simulink model "Missile_Trim"  (R2018b)
settings: Solver=ode4  StartTime=0.0  StopTime=5  FixedStep=Step_Size  RelTol=1e-3  EnableMultiTasking=on
values from neighbouring files (symbols this model uses):
  Alt_Trim = altitude_range(i)    [Missile_Trim_Main.m]    (also in Trim_Solution_a.mat = 0)
  D = 0.150    (= 0.15)    [Missile_Data.m]
  G_Turn = Turn_dot_Trim * Speed_Trim / UNIT_GRAV    [Missile_Trim_Main.m]
  Gamma_Trim = 0.0 * UNIT_DEG2RAD    [Missile_Trim_Main.m]
  Init_Cnstr1 = 0.0    (= 0)    [Missile_Trim_Main.m]
  Init_Cnstr2 = 0.0    (= 0)    [Missile_Trim_Main.m]
  Init_Cnstr3 = 0.0    (= 0)    [Missile_Trim_Main.m]
  Mass = 30.0    (= 30)    [Missile_Data.m]
  S = ( pi / 4 ) * D^2    (= 0.0176714586764)    [Missile_Data.m]
  Speed_Trim = Mach_Trim*interp1(ALT,SOS_Table,Alt_Trim)    [Missile_Trim_Main.m]
  Tbl_ALPHAT = [ 0     4     8    12    16 ]    [Missile_Data.m]
  Tbl_CL_ALPHAT = [ -0.0988   -0.4859   -0.5870   -0.4802   -0.3334   -0.0210 ]    [Missile_Data.m]
  Tbl_CL_DEL_R = [ 5.2712    5.7640    6.1650    6.6234    7.1963    8.4110 ]    [Missile_Data.m]
  Tbl_CL_P = [ -17.9516  -19.6297  -20.9956  -22.5566  -24.5079  -28.6446 ]    [Missile_Data.m]
  Tbl_CM_0 = [ 0   -2.2250   -3.9280   -4.8580   -5.6940 ... (first row only)    [Missile_Data.m]
  Tbl_CM_DEL_P = [ -20.7182  -22.5631  -23.6059  -24.7632  -26.1269  -29.5646 ]    [Missile_Data.m]
  Tbl_CM_PHIT = [ 0   -0.0024   -0.0898   -0.2360   -0.3546 ... (first row only)    [Missile_Data.m]
  Tbl_CM_Q = [ -82.9643  -47.4409  -32.7732  -16.7304  -43.2010  -56.1499 ]    [Missile_Data.m]
  Tbl_CN_DEL_Y = [ -0.3616   -0.3938   -0.4120   -0.4322   -0.4560   -0.5160 ]    [Missile_Data.m]
  Tbl_CN_PHIT = [ 0    0.0040    0.0098    0.1116    0.3049 ... (first row only)    [Missile_Data.m]
  Tbl_CN_R = [ -82.9643  -47.4409  -32.7732  -16.7304  -43.2010  -56.1499 ]    [Missile_Data.m]
  Tbl_CX_0 = [ -0.3840   -0.3670   -0.3550   -0.3460   -0.3390   -0.3410 ]    [Missile_Data.m]
  Tbl_CX_ALPHAT = [ 0.0788    0.0752    0.0680    0.0573    0.0573    0.0573 ]    [Missile_Data.m]
  Tbl_CX_DEL_EFF = [ -16.8080  -17.8585  -18.9090  -19.9595  -20.4847  -23.1110 ]    [Missile_Data.m]
  Tbl_CY_DEL_Y = [ 5.3056    5.7754    6.0504    6.3484    6.6921    7.5745 ]    [Missile_Data.m]
  Tbl_CY_PHIT = [ 0    0.0070    0.0819    0.2313    0.2992 ... (first row only)    [Missile_Data.m]
  Tbl_CZ_0 = [ 0   -2.0680   -3.9700   -5.4250   -6.6810 ... (first row only)    [Missile_Data.m]
  Tbl_CZ_DEL_P = [ -5.3056   -5.7754   -6.0504   -6.3484   -6.6921   -7.5745 ]    [Missile_Data.m]
  Tbl_CZ_PHIT = [ 0    0.0089    0.1842    0.3041    0.2039 ... (first row only)    [Missile_Data.m]
  Tbl_MACH = [ 0.2    0.3    0.4    0.5    0.6    0.7 ]    [Missile_Data.m]
  Theta_dot_Trim = 0.0 * UNIT_DEG2RAD    [Missile_Trim_Main.m]
  Turn_dot_Trim = 0.0 * UNIT_DEG2RAD    [Missile_Trim_Main.m]
  XCG = 0.809    [Missile_Data.m]
  XREF = 0.809    [Missile_Data.m]
undefined symbols (not defined in the file or in its folder): ALT, Init_Euler, Init_Rate, Init_Vel, SOS_Table, UNIT_GRAV
libraries: simulink_extras x6, aerolibtransform2 x4, aerolibasang x3, UAS_Model_library x2, shared6dofsys x2, sharedtransform x1, sharedutil x1, shared6dof x1
settings Model: Creator=e803534  LastModifiedBy=auten
settings OptimizationCC: LifeSpan=inf
settings DebuggingCC: LibraryContextMissingDiagnostic=none  SFUnexpectedBacktrackingDiag=warning  SFNoUnconditionalDefaultTransitionDiag=warning  SFExecutionAtInitializationDiag=none
settings SFSimCC: SimUseLocalCustomCode=off
settings RTWCC: RTWUseLocalCustomCode=off
settings CodeAppCC: StateflowObjectComments=on
settings GRTTargetCC: TargetLangStandard=C89/C90 (ANSI)  GeneratePreprocessorConditionals=Disable all
settings ConfigComp: CovMetricSettings=dw  CovHtmlReporting=on  CovSaveCumulativeToWorkspaceVar=on  CovSaveSingleToWorkspaceVar=on  CovExternalEMLEnable=off

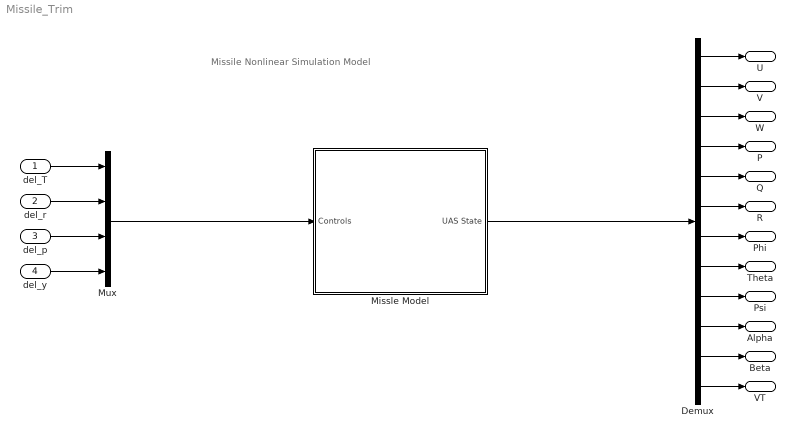
== system Missile_Trim ==
  note: Missile Nonlinear Simulation Model
  del_T : Inport
  "del_r " : Inport  Port=2
  del_p : Inport  Port=3
  del_y : Inport  Port=4
  Demux : Demux  Outputs=12
  Missle Model : Subsystem
  Mux : Mux
  U : Outport
  V : Outport  Port=2
  W : Outport  Port=3
  P : Outport  Port=4
  Q : Outport  Port=5
  R : Outport  Port=6
  Phi : Outport  Port=7
  Theta : Outport  Port=8
  Psi : Outport  Port=9
  Alpha : Outport  Port=10
  Beta : Outport  Port=11
  VT : Outport  Port=12
  wires:
  Mux/1 -> Missle Model/1(Controls)
  del_p/1 -> Mux/3
  "del_r "/1 -> Mux/2
  del_T/1 -> Mux/1
  del_y/1 -> Mux/4
  Missle Model/1(UAS State) -> Demux/1
  Demux/1 -> U/1
  Demux/3 -> W/1
  Demux/5 -> Q/1
  Demux/6 -> R/1
  Demux/7 -> Phi/1
  Demux/9 -> Psi/1
  Demux/10 -> Alpha/1
  Demux/11 -> Beta/1
  Demux/12 -> VT/1
  Demux/4 -> P/1
  Demux/2 -> V/1
  Demux/8 -> Theta/1

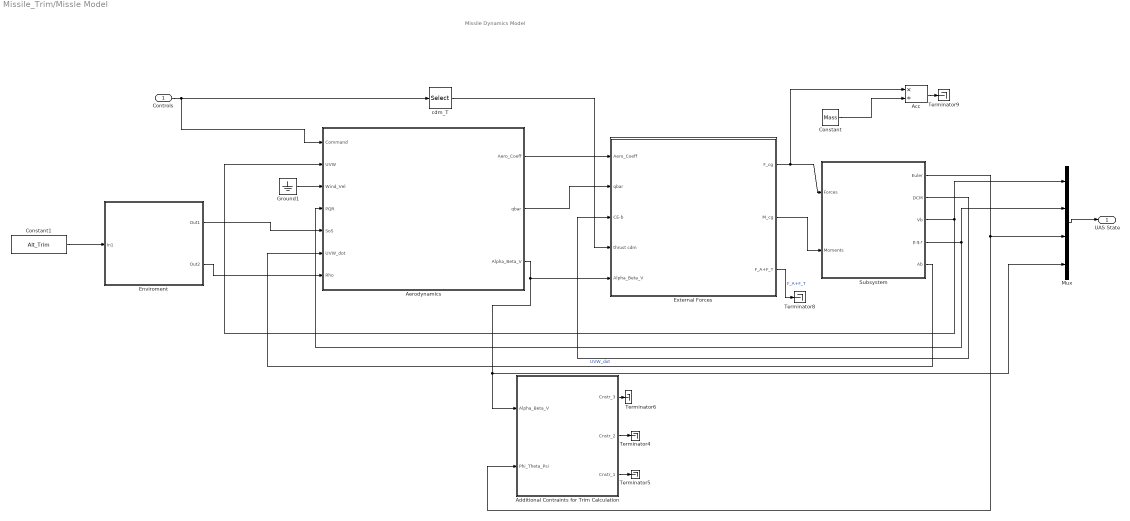
== system Missile_Trim/Missle Model ==
  note: Missile Dynamics Model
  Controls : Inport
  Acc : Product  Inputs=*/  RndMeth=Zero
  Additional Contraints for Trim Calculation : Subsystem
  Aerodynamics : Subsystem
  Constant : Constant  Value=Mass
  Constant1 : Constant  Value=Alt_Trim
  Enviroment : Subsystem
  External Forces : Subsystem
  Ground1 : Ground
  Mux : Mux
  Subsystem : Subsystem
  Terminator{4..6,8..9} (5 alike) : Terminator
  cdm_T : Selector  InputPortWidth=4  IndexOptions=Index vector (dialog)  Indices=[1]  OutputSizes=1
  UAS State : Outport
  wires:
  Controls/1 -> Aerodynamics/1(Command), cdm_T/1
  External Forces/1(F_cg) -> Subsystem/1(Forces), Acc/1
  External Forces/2(M_cg) -> Subsystem/2(Moments)
  Constant/1 -> Acc/2
  Mux/1 -> UAS State/1
  Subsystem/3(Vb) -> Mux/1, Aerodynamics/2(UVW)
  Subsystem/4(p,q,r) -> Aerodynamics/4(PQR), Mux/2
  Acc/1 -> Terminator9/1
  Additional Contraints for Trim Calculation/2(Cnstr_2) -> Terminator4/1
  Additional Contraints for Trim Calculation/3(Cnstr_1) -> Terminator5/1
  Additional Contraints for Trim Calculation/1(Cnstr_3) -> Terminator6/1
  Subsystem/1(Euler) -> Mux/3, Additional Contraints for Trim Calculation/2(Phi_Theta_Psi)
  Subsystem/2(DCM) -> External Forces/3(CE-b)
  cdm_T/1 -> External Forces/4(thrust cdm)
  External Forces/3(F_A+F_T) -> Terminator8/1  "F_A+F_T"
  Aerodynamics/3(Alpha_Beta_V) -> Additional Contraints for Trim Calculation/1(Alpha_Beta_V), Mux/4, External Forces/5(Alpha_Beta_V)
  Ground1/1 -> Aerodynamics/3(Wind_Vel)
  Subsystem/5(Ab) -> Aerodynamics/6(UVW_dot)  "UVW_dot"
  Aerodynamics/1(Aero_Coeff) -> External Forces/1(Aero_Coeff)
  Aerodynamics/2(qbar) -> External Forces/2(qbar)
  Constant1/1 -> Enviroment/1(In1)
  Enviroment/1(Out1) -> Aerodynamics/5(SoS)
  Enviroment/2(Out2) -> Aerodynamics/7(Rho)

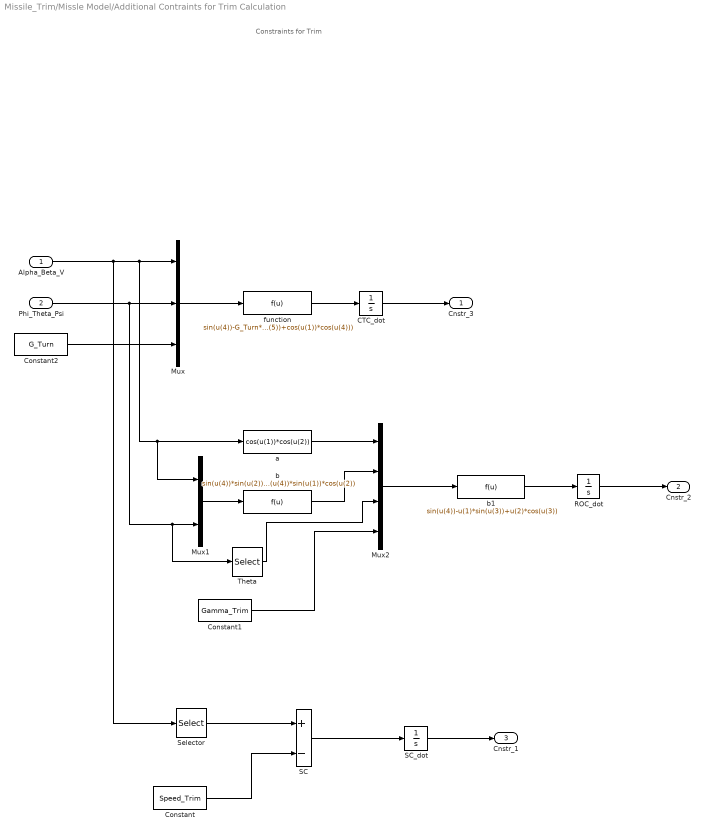
== system Missile_Trim/Missle Model/Additional Contraints for Trim Calculation ==
  note: Constraints for Trim
  Alpha_Beta_V : Inport  PortDimensions=3
  Phi_Theta_Psi : Inport  Port=2  PortDimensions=3
  CTC_dot : Integrator  InitialCondition=Init_Cnstr3
  Constant : Constant  Value=Speed_Trim
  Constant1 : Constant  Value=Gamma_Trim
  Constant2 : Constant  Value=G_Turn
  Mux : Mux  Inputs=3
  Mux1 : Mux  Inputs=2
  Mux2 : Mux
  ROC_dot : Integrator  InitialCondition=Init_Cnstr2
  SC : Sum  Inputs=+-
  SC_dot : Integrator  InitialCondition=Init_Cnstr1
  Selector : Selector  InputPortWidth=3  IndexOptions=Index vector (dialog)  Indices=[3]  OutputSizes=1
  Theta : Selector  InputPortWidth=3  IndexOptions=Index vector (dialog)  Indices=[2]  OutputSizes=1
  a : Fcn  Expr=cos(u(1))*cos(u(2))
  b : Fcn  Expr=sin(u(4))*sin(u(2))+cos(u(4))*sin(u(1))*cos(u(2))
  b1 : Fcn  Expr=sin(u(4))-u(1)*sin(u(3))+u(2)*cos(u(3))
  function : Fcn  Expr=sin(u(4))-G_Turn*cos(u(2))*(sin(u(1))*tan(u(5))+cos(u(1))*cos(u(4)))
  Cnstr_3 : Outport
  Cnstr_2 : Outport  Port=2
  Cnstr_1 : Outport  Port=3
  wires:
  CTC_dot/1 -> Cnstr_3/1
  Alpha_Beta_V/1 -> Selector/1, Mux1/1, a/1, Mux/1
  Phi_Theta_Psi/1 -> Theta/1, Mux1/2, Mux/2
  Constant2/1 -> Mux/3
  Mux/1 -> function/1
  function/1 -> CTC_dot/1
  Mux1/1 -> b/1
  b/1 -> Mux2/2
  a/1 -> Mux2/1
  Constant1/1 -> Mux2/4
  Theta/1 -> Mux2/3
  Mux2/1 -> b1/1
  ROC_dot/1 -> Cnstr_2/1
  b1/1 -> ROC_dot/1
  SC_dot/1 -> Cnstr_1/1
  Selector/1 -> SC/1
  Constant/1 -> SC/2
  SC/1 -> SC_dot/1

== system Missile_Trim/Missle Model/Aerodynamics ==
  Command : Inport
  UVW : Inport  Port=2
  Wind_Vel : Inport  Port=3
  PQR : Inport  Port=4
  SoS : Inport  Port=5
  UVW_dot : Inport  Port=6
  Rho : Inport  Port=7
  Aerodynanamic Coefficents : Subsystem
  Wind-axes Velocitie : Subsystem  AncestorBlock=UAS_Model_library/External Forces/Aerodynamics/Wind-axes Velocitie
  Aero_Coeff : Outport
  qbar : Outport  Port=2
  Alpha_Beta_V : Outport  Port=3
  wires:
  SoS/1 -> Wind-axes Velocitie/3(SoS)
  UVW/1 -> Wind-axes Velocitie/1(UVW)
  Aerodynanamic Coefficents/1(Aero_Coeff) -> Aero_Coeff/1
  Wind-axes Velocitie/1(Alpha_Beta_V) -> Alpha_Beta_V/1, Aerodynanamic Coefficents/2(Alpha_Beta_V)  "Alpha_Beta_V"
  Wind-axes Velocitie/3(qbar) -> qbar/1
  Wind-axes Velocitie/2(Mach) -> Aerodynanamic Coefficents/3(Mach)
  UVW_dot/1 -> Wind-axes Velocitie/5(UVW_dot)
  PQR/1 -> Aerodynanamic Coefficents/4(PQR), Wind-axes Velocitie/6(PQR)
  Rho/1 -> Wind-axes Velocitie/4(Rho)
  Wind_Vel/1 -> Wind-axes Velocitie/2(Wind_Vel)
  Command/1 -> Aerodynanamic Coefficents/1(Command)

== system Missile_Trim/Missle Model/Enviroment ==
  In1 : Inport
  1-D Lookup Table : Lookup_n-D  NumberOfTableDimensions=1  BreakpointsForDimension1=ALT  Table=SOS_Table  InternalRulePriority=Speed  RndMeth=Simplest  InputSameDT=on
  Atmosphere Model : UAS_Model_library/Envrionment/Atmosphere Model  SystemSampleTime=-1
  Terminator2 : Terminator
  Out1 : Outport
  Out2 : Outport  Port=2
  wires:
  In1/1 -> Atmosphere Model/1, 1-D Lookup Table/1
  Atmosphere Model/1 -> Terminator2/1
  Atmosphere Model/2 -> Out2/1
  1-D Lookup Table/1 -> Out1/1

== system Missile_Trim/Missle Model/External Forces ==
  Aero_Coeff : Inport
  qbar : Inport  Port=2
  CE-b : Inport  Port=3
  thrust cdm : Inport  Port=4
  Alpha_Beta_V : Inport  Port=5
  Aerodynamic Force & Moment : Subsystem  AncestorBlock=UAS_Model_library/External Forces/Aerodynamics/Aerodynamic Force & Moment
  Propulsive Force & Moment : Subsystem  AncestorBlock=UAS_Model_library/External Forces/Propulsive/Propulsive Force & Moment
  Sum of Aerodynamic and Propulsion Forces : Sum
  Total Force & Moment : Subsystem  AncestorBlock=UAS_Model_library/External Forces/Total Force & Moment
  F_cg : Outport
  M_cg : Outport  Port=2
  F_A+F_T : Outport  Port=3
  wires:
  Total Force & Moment/2(M_cg) -> M_cg/1
  Aerodynamic Force & Moment/2(M_aero) -> Total Force & Moment/2(M_aero)
  Propulsive Force & Moment/2(M_prop) -> Total Force & Moment/4(M_prop)
  Total Force & Moment/1(F_cg) -> F_cg/1
  Aerodynamic Force & Moment/1(F_aero) -> Sum of Aerodynamic and Propulsion Forces/1, Total Force & Moment/1(F_aero)
  Propulsive Force & Moment/1(F_prop) -> Sum of Aerodynamic and Propulsion Forces/2, Total Force & Moment/3(F_prop)
  qbar/1 -> Aerodynamic Force & Moment/2(qbar)
  Aero_Coeff/1 -> Aerodynamic Force & Moment/1(Aero_Coeff)
  Sum of Aerodynamic and Propulsion Forces/1 -> F_A+F_T/1
  CE-b/1 -> Total Force & Moment/5("cE-B ")
  thrust cdm/1 -> Propulsive Force & Moment/1(Controls)
  Alpha_Beta_V/1 -> ?

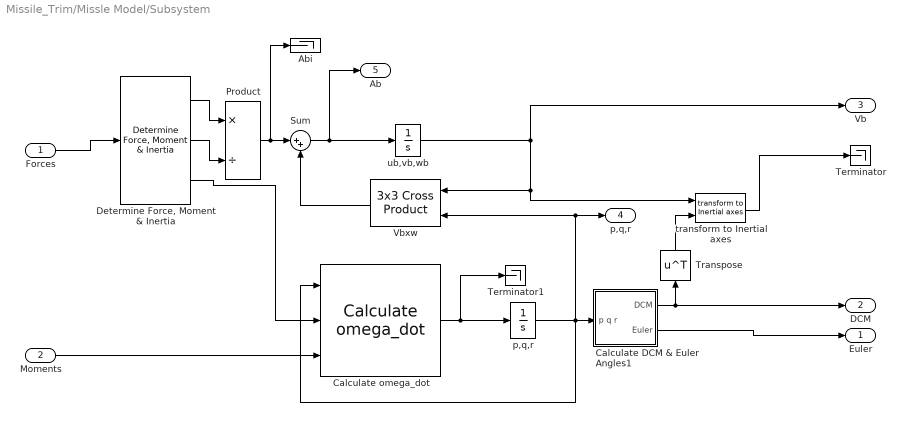
== system Missile_Trim/Missle Model/Subsystem ==
  Forces : Inport  Unit=N  PortDimensions=3
  Moments : Inport  Port=2  Unit=N*m  PortDimensions=3
  Abi : Terminator
  Calculate DCM & Euler Angles1 : Subsystem
  Calculate omega_dot : shared6dofsys/Calculate omega_dot  aMode=aMode
      settings: SourceProductName=Aerospace Blockset  SourceProductBaseCode=AE
  "Determine Force, Moment & Inertia" : UAS_Model_library/Equations of Motion/Determine Force, Moment & Inertia  SystemSampleTime=-1
  Product : Product  Inputs=*/  SaturateOnIntegerOverflow=on  OutDataTypeStr=Inherit: Same as first input
  Sum : Sum  Inputs=|++  SaturateOnIntegerOverflow=on
  Terminator : Terminator
  Terminator1 : Terminator
  Transpose : Math  Operator=transpose  SaturateOnIntegerOverflow=on
  Vbxw : sharedutil/3x3 Cross Product  aMode=aMode
      settings: SourceProductBaseCode=AE
  "p,q,r " : Integrator  InitialCondition=Init_Rate
  "transform to Inertial axes " : shared6dof/6DOF (Euler Angles)/transform to Inertial axes   SystemSampleTime=-1
      settings: SourceProductName=Aerospace Blockset  SourceProductBaseCode=AE
  ub,vb,wb : Integrator  InitialCondition=Init_Vel
  Euler : Outport  Unit=rad
  DCM : Outport  Port=2  Unit=1
  Vb : Outport  Port=3  Unit=m/s
  p,q,r : Outport  Port=4  Unit=rad/s
  Ab : Outport  Port=5  Unit=m/s^2
  wires:
  "transform to Inertial axes "/1 -> Terminator/1
  Calculate omega_dot/1 -> Terminator1/1, "p,q,r "/1
  Sum/1 -> ub,vb,wb/1, Ab/1
  Vbxw/1 -> Sum/2
  Product/1 -> Sum/1, Abi/1
  "p,q,r "/1 -> Calculate DCM & Euler Angles1/1("p q r "), Calculate omega_dot/1, p,q,r/1, Vbxw/2
  Forces/1 -> "Determine Force, Moment & Inertia"/1
  ub,vb,wb/1 -> Vb/1, "transform to Inertial axes "/1, Vbxw/1
  "Determine Force, Moment & Inertia"/2 -> Product/2
  Moments/1 -> Calculate omega_dot/3
  Calculate DCM & Euler Angles1/2(Euler) -> Euler/1
  Calculate DCM & Euler Angles1/1(DCM) -> Transpose/1, DCM/1
  "Determine Force, Moment & Inertia"/3 -> Calculate omega_dot/2
  Transpose/1 -> "transform to Inertial axes "/2
  "Determine Force, Moment & Inertia"/1 -> Product/1

== system Missile_Trim/Missle Model/Aerodynamics/Aerodynanamic Coefficents ==
  Command : Inport
  Alpha_Beta_V : Inport  Port=2
  Mach : Inport  Port=3
  PQR : Inport  Port=4
  Aerodynamics : Subsystem
  del_r del_p del_y : Selector  InputPortWidth=4  IndexOptions=Index vector (dialog)  Indices=[2 3 4]  OutputSizes=1
  delta_eff : Subsystem
  total angle of AoA and Roll : Subsystem
  Aero_Coeff : Outport
  wires:
  del_r del_p del_y/1 -> Aerodynamics/3(control inputs), delta_eff/1(controll)
  total angle of AoA and Roll/2(phi_t) -> Aerodynamics/5(phi_t)
  delta_eff/1(delta_eff) -> Aerodynamics/2(delta_eff)
  Alpha_Beta_V/1 -> total angle of AoA and Roll/1(alpha_beta_V), Aerodynamics/6(alpha_beta_V)
  Command/1 -> del_r del_p del_y/1
  total angle of AoA and Roll/1(alpha_t) -> Aerodynamics/4(alpha_t)
  PQR/1 -> Aerodynamics/7(PQR)
  Aerodynamics/1(Aero_Coeff) -> Aero_Coeff/1
  Mach/1 -> Aerodynamics/1(Mach Number)

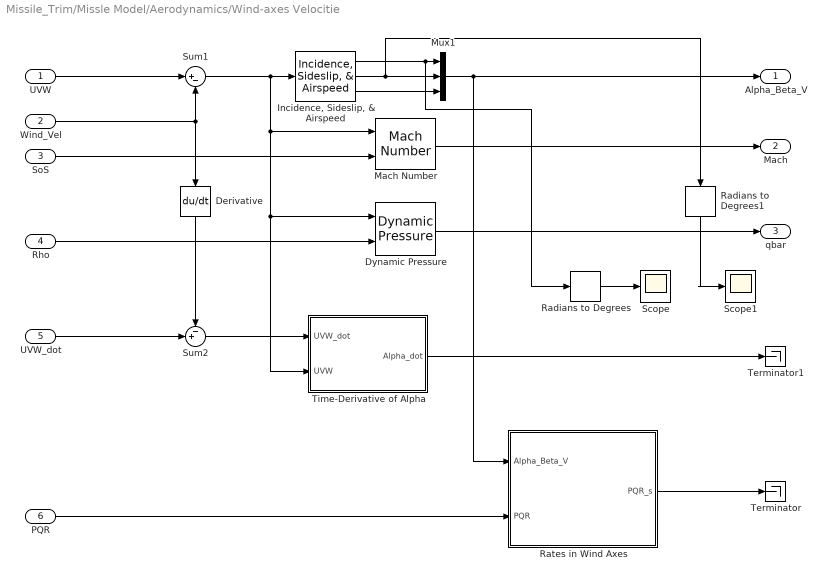
== system Missile_Trim/Missle Model/Aerodynamics/Wind-axes Velocitie ==
  UVW : Inport
  Wind_Vel : Inport  Port=2
  SoS : Inport  Port=3
  Rho : Inport  Port=4
  UVW_dot : Inport  Port=5
  PQR : Inport  Port=6
  Derivative : Derivative
  Dynamic Pressure : aerolibasang/Dynamic Pressure
  "Incidence, Sideslip, & Airspeed" : aerolibasang/Incidence, Sideslip, & Airspeed
      settings: SourceProductName=Aerospace Blockset
  Mach Number : aerolibasang/Mach Number
      settings: SourceProductName=Aerospace Blockset  SourceProductBaseCode=AE
  Mux1 : Mux  Inputs=3
  Radians to Degrees : simulink_extras/Transformations/Radians to Degrees
  Radians to Degrees1 : simulink_extras/Transformations/Radians to Degrees
  Rates in Wind Axes : Subsystem
  Scope : Scope
  Scope1 : Scope
  Sum1 : Sum  Inputs=|+-  SaturateOnIntegerOverflow=on  InputSameDT=on  OutDataTypeStr=Inherit: Same as first input
  Sum2 : Sum  Inputs=-+|  SaturateOnIntegerOverflow=on  InputSameDT=on  OutDataTypeStr=Inherit: Same as first input
  Terminator : Terminator
  Terminator1 : Terminator
  Time-Derivative of Alpha : Subsystem
  Alpha_Beta_V : Outport
  Mach : Outport  Port=2
  qbar : Outport  Port=3
  wires:
  PQR/1 -> Rates in Wind Axes/2(PQR)
  Rates in Wind Axes/1(PQR_s) -> Terminator/1
  "Incidence, Sideslip, & Airspeed"/3 -> Mux1/3
  "Incidence, Sideslip, & Airspeed"/2 -> Radians to Degrees1/1, Mux1/2
  "Incidence, Sideslip, & Airspeed"/1 -> Radians to Degrees/1, Mux1/1
  Sum1/1 -> "Incidence, Sideslip, & Airspeed"/1, Mach Number/1, Dynamic Pressure/1, Time-Derivative of Alpha/2(UVW)
  Mux1/1 -> Alpha_Beta_V/1, Rates in Wind Axes/1(Alpha_Beta_V)
  UVW/1 -> Sum1/1
  Wind_Vel/1 -> Derivative/1, Sum1/2
  Mach Number/1 -> Mach/1
  SoS/1 -> Mach Number/2
  Rho/1 -> Dynamic Pressure/2
  Dynamic Pressure/1 -> qbar/1
  Time-Derivative of Alpha/1(Alpha_dot) -> Terminator1/1
  UVW_dot/1 -> Sum2/2
  Sum2/1 -> Time-Derivative of Alpha/1(UVW_dot)
  Derivative/1 -> Sum2/1
  Radians to Degrees/1 -> Scope/1
  Radians to Degrees1/1 -> Scope1/1

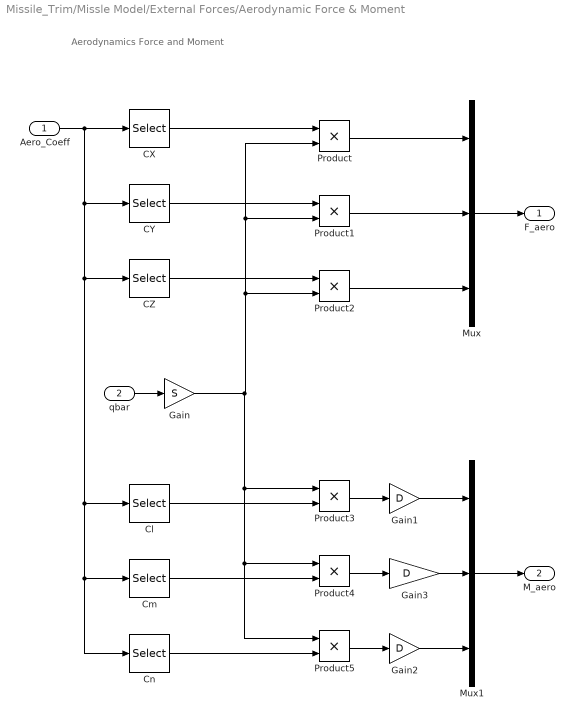
== system Missile_Trim/Missle Model/External Forces/Aerodynamic Force & Moment ==
  note: Aerodynamics Force and Moment
  Aero_Coeff : Inport
  qbar : Inport  Port=2
  CX : Selector  InputPortWidth=6  IndexOptions=Index vector (dialog)  Indices=[1]  OutputSizes=1
  CY : Selector  InputPortWidth=6  IndexOptions=Index vector (dialog)  Indices=[2]  OutputSizes=1
  CZ : Selector  InputPortWidth=6  IndexOptions=Index vector (dialog)  Indices=[3]  OutputSizes=1
  Cl : Selector  InputPortWidth=6  IndexOptions=Index vector (dialog)  Indices=[4]  OutputSizes=1
  Cm : Selector  InputPortWidth=6  IndexOptions=Index vector (dialog)  Indices=[5]  OutputSizes=1
  Cn : Selector  InputPortWidth=6  IndexOptions=Index vector (dialog)  Indices=[6]  OutputSizes=1
  Gain : Gain  Gain=S
  Gain1 : Gain  Gain=D
  Gain2 : Gain  Gain=D
  Gain3 : Gain  Gain=D
  Mux : Mux  Inputs=3
  Mux1 : Mux  Inputs=3
  Product{,1..5} (6 alike) : Product
  F_aero : Outport
  M_aero : Outport  Port=2
  wires:
  Gain3/1 -> Mux1/2
  Gain2/1 -> Mux1/3
  Gain1/1 -> Mux1/1
  Mux1/1 -> M_aero/1
  Product5/1 -> Gain2/1
  Product4/1 -> Gain3/1
  Product3/1 -> Gain1/1
  Cn/1 -> Product5/2
  Cm/1 -> Product4/2
  Cl/1 -> Product3/2
  Mux/1 -> F_aero/1
  Product2/1 -> Mux/3
  Product1/1 -> Mux/2
  Product/1 -> Mux/1
  CZ/1 -> Product2/1
  CY/1 -> Product1/1
  Gain/1 -> Product/2, Product1/2, Product2/2, Product3/1, Product4/1, Product5/1
  CX/1 -> Product/1
  qbar/1 -> Gain/1
  Aero_Coeff/1 -> CX/1, CY/1, CZ/1, Cm/1, Cn/1, Cl/1

== system Missile_Trim/Missle Model/External Forces/Propulsive Force & Moment ==
  note: Propulsive Force and Moment
  Controls : Inport
  Constant : Constant  Value=0
  Mux : Mux  Inputs=3
  Mux1 : Mux  Inputs=3
  F_prop : Outport
  M_prop : Outport  Port=2
  wires:
  Mux/1 -> F_prop/1
  Controls/1 -> Mux/1
  Constant/1 -> Mux/2, Mux1/1, Mux1/2, Mux1/3, Mux/3
  Mux1/1 -> M_prop/1

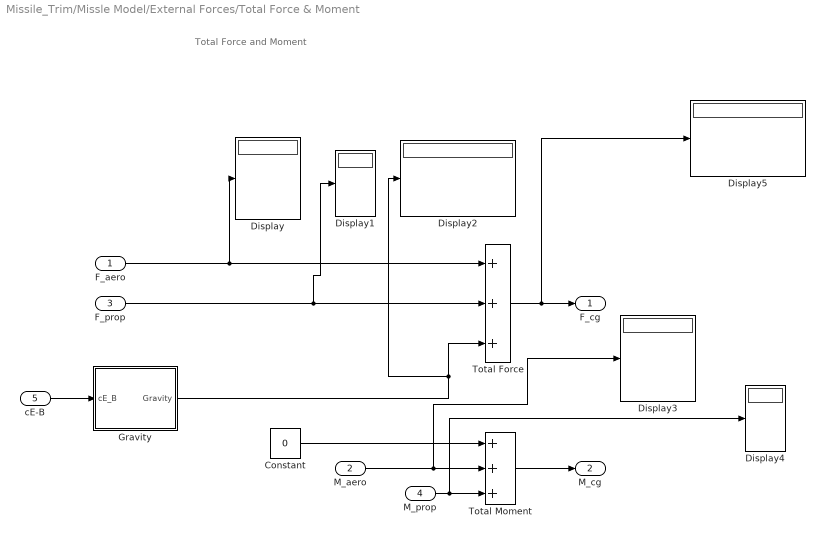
== system Missile_Trim/Missle Model/External Forces/Total Force & Moment ==
  note: Total Force and Moment
  F_aero : Inport  PortDimensions=3
  M_aero : Inport  Port=2  PortDimensions=3
  F_prop : Inport  Port=3  PortDimensions=3
  M_prop : Inport  Port=4  PortDimensions=3
  "cE-B " : Inport  Port=5
  Constant : Constant  Value=0
  Display{,1..5} (6 alike) : Display
  Gravity : Subsystem  AncestorBlock=UAS_Model_library/Envrionment/Gravity
  Total Force : Sum  Inputs=+++  SaturateOnIntegerOverflow=on  InputSameDT=on  OutDataTypeStr=Inherit: Same as first input
  Total Moment : Sum  Inputs=+++  SaturateOnIntegerOverflow=on  InputSameDT=on  OutDataTypeStr=Inherit: Same as first input
  F_cg : Outport
  M_cg : Outport  Port=2
  wires:
  Gravity/1(Gravity) -> Total Force/3, Display2/1
  Total Moment/1 -> M_cg/1
  M_prop/1 -> Display4/1, Total Moment/3
  F_prop/1 -> Display1/1, Total Force/2
  F_aero/1 -> Display/1, Total Force/1
  Constant/1 -> Total Moment/1
  M_aero/1 -> Display3/1, Total Moment/2
  "cE-B "/1 -> Gravity/1(cE_B)
  Total Force/1 -> Display5/1, F_cg/1

== system Missile_Trim/Missle Model/Subsystem/Calculate DCM & Euler Angles1 ==
  "p q r " : Inport
  Constant : Constant  Value=Theta_dot_Trim
  Constant1 : Constant  Value=Turn_dot_Trim
  Demux : Demux  Outputs=3
  Mux : Mux  Inputs=3
  Rotation Angles to Direction Cosine Matrix : sharedtransform/Rotation Angles to Direction Cosine Matrix  rotationOrder=ZYX  aMode=aMode
      settings: SourceProductBaseCode=AE
  Selector : Selector  InputPortWidth=3  IndexOptions=Index vector (dialog)  Indices=[3 2 1]  OutputSizes=1
  Sum : Sum  Inputs=|+-
  Sum1 : Sum  Inputs=|+-
  phi theta psi : Integrator  InitialCondition=Init_Euler
  phidot thetadot psidot : shared6dofsys/DCM & Euler Angles (Euler)/phidot thetadot psidot  SystemSampleTime=-1
      settings: SourceProductName=Aerospace Blockset  SourceProductBaseCode=AE
  DCM : Outport
  Euler : Outport  Port=2
  wires:
  Selector/1 -> Rotation Angles to Direction Cosine Matrix/1
  phi theta psi/1 -> Euler/1, Selector/1, phidot thetadot psidot/2
  "p q r "/1 -> phidot thetadot psidot/1
  Rotation Angles to Direction Cosine Matrix/1 -> DCM/1
  phidot thetadot psidot/1 -> Demux/1
  Mux/1 -> phi theta psi/1
  Sum/1 -> Mux/2
  Sum1/1 -> Mux/3
  Constant/1 -> Sum/2
  Constant1/1 -> Sum1/2
  Demux/3 -> Sum1/1
  Demux/2 -> Sum/1
  Demux/1 -> Mux/1

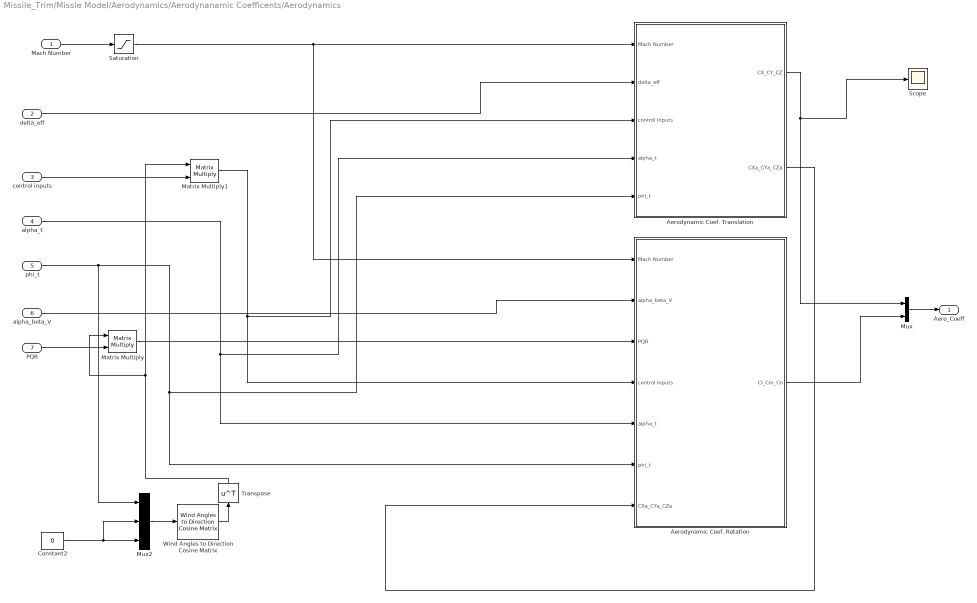
== system Missile_Trim/Missle Model/Aerodynamics/Aerodynanamic Coefficents/Aerodynamics ==
  Mach Number : Inport
  delta_eff : Inport  Port=2
  control inputs : Inport  Port=3
  alpha_t : Inport  Port=4
  phi_t : Inport  Port=5
  alpha_beta_V : Inport  Port=6
  PQR : Inport  Port=7
  Aerodynamic Coef. Rotation : Subsystem
  Aerodynamic Coef. Translation : Subsystem
  Constant2 : Constant  Value=0
  Matrix Multiply : Product  Multiplication=Matrix(*)
  Matrix Multiply1 : Product  Multiplication=Matrix(*)
  Mux : Mux  Inputs=2
  Mux2 : Mux  Inputs=3
  Saturation : Saturate  UpperLimit=0.7  LowerLimit=0.2
  Scope : Scope
  Transpose : Math  Operator=transpose  SaturateOnIntegerOverflow=on
  Wind Angles to Direction Cosine Matrix : aerolibtransform2/Wind Angles to  Direction Cosine Matrix
      settings: SourceProductName=Aerospace Blockset  SourceProductBaseCode=AE
  Aero_Coeff : Outport
  wires:
  Aerodynamic Coef. Translation/2(CXa_CYa_CZa) -> Aerodynamic Coef. Rotation/7(CXa_CYa_CZa)
  Mach Number/1 -> Saturation/1
  delta_eff/1 -> Aerodynamic Coef. Translation/2(delta_eff)
  Matrix Multiply1/1 -> Aerodynamic Coef. Rotation/4(control inputs), Aerodynamic Coef. Translation/3(control inputs)
  alpha_beta_V/1 -> Aerodynamic Coef. Rotation/2(alpha_beta_V)
  Matrix Multiply/1 -> Aerodynamic Coef. Rotation/3(PQR)
  Aerodynamic Coef. Translation/1(CX_CY_CZ) -> Scope/1, Mux/1
  Aerodynamic Coef. Rotation/1(Cl_Cm_Cn) -> Mux/2
  Mux/1 -> Aero_Coeff/1
  alpha_t/1 -> Aerodynamic Coef. Rotation/5(alpha_t), Aerodynamic Coef. Translation/4(alpha_t)
  phi_t/1 -> Mux2/1, Aerodynamic Coef. Translation/5(phi_t), Aerodynamic Coef. Rotation/6(phi_t)
  Mux2/1 -> Wind Angles to Direction Cosine Matrix/1
  Constant2/1 -> Mux2/2, Mux2/3
  control inputs/1 -> Matrix Multiply1/2
  Wind Angles to Direction Cosine Matrix/1 -> Transpose/1
  PQR/1 -> Matrix Multiply/2
  Transpose/1 -> Matrix Multiply/1, Matrix Multiply1/1
  Saturation/1 -> Aerodynamic Coef. Rotation/1(Mach Number), Aerodynamic Coef. Translation/1(Mach Number)

== system Missile_Trim/Missle Model/Aerodynamics/Aerodynanamic Coefficents/delta_eff ==
  controll : Inport
  Abs : Abs
  Abs1 : Abs
  Constant : Constant  Value=2
  Divide : Product  Inputs=*/  SaturateOnIntegerOverflow=on  RndMeth=Zero
  Selector : Selector  InputPortWidth=3  IndexOptions=Index vector (dialog)  Indices=[3]  OutputSizes=1
  Selector1 : Selector  InputPortWidth=3  IndexOptions=Index vector (dialog)  Indices=[2]  OutputSizes=1
  Sum : Sum  Inputs=|++
  delta_eff : Outport
  wires:
  Selector1/1 -> Abs1/1
  Sum/1 -> Divide/1
  Constant/1 -> Divide/2
  Divide/1 -> delta_eff/1
  controll/1 -> Selector/1, Selector1/1
  Selector/1 -> Abs/1
  Abs/1 -> Sum/1
  Abs1/1 -> Sum/2

== system Missile_Trim/Missle Model/Aerodynamics/Aerodynanamic Coefficents/total angle of AoA and Roll ==
  alpha_beta_V : Inport
  Asin : Trigonometry  Operator=acos
  Atan2 : Trigonometry  Operator=atan2
  Cos : Trigonometry  Operator=cos
  Cos1 : Trigonometry  Operator=cos
  Multiply : Product
  Selector : Selector  InputPortWidth=3  IndexOptions=Index vector (dialog)  Indices=[1]  OutputSizes=1
  Selector1 : Selector  InputPortWidth=3  IndexOptions=Index vector (dialog)  Indices=[2]  OutputSizes=1
  Sin : Trigonometry
  Tan : Trigonometry  Operator=tan
  alpha_t : Outport
  phi_t : Outport  Port=2
  wires:
  Sin/1 -> Atan2/2
  Tan/1 -> Atan2/1
  Selector/1 -> Sin/1, Cos/1
  Selector1/1 -> Tan/1, Cos1/1
  Cos1/1 -> Multiply/2
  Multiply/1 -> Asin/1
  Cos/1 -> Multiply/1
  Atan2/1 -> phi_t/1
  Asin/1 -> alpha_t/1
  alpha_beta_V/1 -> Selector1/1, Selector/1

== system Missile_Trim/Missle Model/Aerodynamics/Wind-axes Velocitie/Rates in Wind Axes ==
  note: Rates in Wind Axes
  Alpha_Beta_V : Inport
  PQR : Inport  Port=2
  Alpha : Selector  InputPortWidth=3  IndexOptions=Index vector (dialog)  Indices=[1]  OutputSizes=1
  Beta_Ref : Constant  Value=0
  Direction Cosine Matrix Body to Wind : aerolibtransform2/Direction Cosine Matrix Body to Wind
      settings: SourceProductName=Aerospace Blockset  SourceProductBaseCode=AE
  Mux : Mux  Inputs=2
  transform to body axes : Product  Inputs=**  Multiplication=Matrix(*)  SaturateOnIntegerOverflow=on  InputSameDT=on  OutDataTypeStr=Inherit: Same as first input
  PQR_s : Outport
  wires:
  Beta_Ref/1 -> Mux/2
  Mux/1 -> Direction Cosine Matrix Body to Wind/1
  transform to body axes/1 -> PQR_s/1
  PQR/1 -> transform to body axes/2
  Direction Cosine Matrix Body to Wind/1 -> transform to body axes/1  "cB_W"
  Alpha/1 -> Mux/1
  Alpha_Beta_V/1 -> Alpha/1

== system Missile_Trim/Missle Model/Aerodynamics/Wind-axes Velocitie/Time-Derivative of Alpha ==
  note: Time Derivative of Alpha
  UVW_dot : Inport
  UVW : Inport  Port=2
  Add : Sum  Inputs=-+
  Add1 : Sum
  Demux2 : Demux  Outputs=3
  Demux3 : Demux  Outputs=3
  Divide : Product  Inputs=*/
  Math Function2 : Math  Operator=square  SaturateOnIntegerOverflow=on
  Math Function3 : Math  Operator=square  SaturateOnIntegerOverflow=on
  Product3 : Product
  Product4 : Product
  Terminator2 : Terminator
  Terminator3 : Terminator
  Alpha_dot : Outport
  wires:
  Divide/1 -> Alpha_dot/1
  Add1/1 -> Divide/2
  Math Function3/1 -> Add1/2
  Math Function2/1 -> Add1/1
  Add/1 -> Divide/1
  Product3/1 -> Add/1
  Product4/1 -> Add/2
  Demux3/1 -> Product4/2, Math Function2/1
  Demux2/3 -> Product4/1
  Demux3/3 -> Product3/2, Math Function3/1
  Demux3/2 -> Terminator3/1
  UVW/1 -> Demux3/1
  Demux2/1 -> Product3/1
  Demux2/2 -> Terminator2/1
  UVW_dot/1 -> Demux2/1

== system Missile_Trim/Missle Model/External Forces/Total Force & Moment/Gravity ==
  cE_B : Inport
  Constant : Constant  Value=0
  Constant1 : Constant  Value=Mass
  Display : Display
  Display1 : Display
  "Gravity vector in body frame " : Product  Multiplication=Matrix(*)  SaturateOnIntegerOverflow=on  InputSameDT=on  OutDataTypeStr=Inherit: Same as first input
  Mux1 : Mux  Inputs=3
  g : Gain  Gain=UNIT_GRAV
  Gravity : Outport
  wires:
  Constant1/1 -> g/1
  "Gravity vector in body frame "/1 -> Display/1, Gravity/1
  g/1 -> Mux1/3
  Mux1/1 -> "Gravity vector in body frame "/2
  cE_B/1 -> Display1/1, "Gravity vector in body frame "/1
  Constant/1 -> Mux1/1, Mux1/2

== system Missile_Trim/Missle Model/Aerodynamics/Aerodynanamic Coefficents/Aerodynamics/Aerodynamic Coef. Rotation ==
  Mach Number : Inport
  alpha_beta_V : Inport  Port=2
  PQR : Inport  Port=3
  control inputs : Inport  Port=4
  alpha_t : Inport  Port=5
  phi_t : Inport  Port=6
  CXa_CYa_CZa : Inport  Port=7
  Constant2 : Constant  Value=0
  Matrix Multiply : Product  Multiplication=Matrix(*)
  Mux : Mux  Inputs=3
  Mux2 : Mux  Inputs=3
  Subsystem Aero. Coef. Rotation : Subsystem
  Wind Angles to Direction Cosine Matrix : aerolibtransform2/Wind Angles to  Direction Cosine Matrix
      settings: SourceProductName=Aerospace Blockset  SourceProductBaseCode=AE
  Cl_Cm_Cn : Outport
  wires:
  Mux/1 -> Matrix Multiply/2
  Matrix Multiply/1 -> Cl_Cm_Cn/1
  Mach Number/1 -> Subsystem Aero. Coef. Rotation/1(Mach Number)
  alpha_beta_V/1 -> Subsystem Aero. Coef. Rotation/4(alpha_beta_V)
  PQR/1 -> Subsystem Aero. Coef. Rotation/5(PQR)
  control inputs/1 -> Subsystem Aero. Coef. Rotation/6(control)
  alpha_t/1 -> Subsystem Aero. Coef. Rotation/2(alpha_t)
  phi_t/1 -> Mux2/1, Subsystem Aero. Coef. Rotation/3(phi_t)
  CXa_CYa_CZa/1 -> Subsystem Aero. Coef. Rotation/7(C_X_C_Y_CZ)
  Mux2/1 -> Wind Angles to Direction Cosine Matrix/1
  Constant2/1 -> Mux2/2, Mux2/3
  Wind Angles to Direction Cosine Matrix/1 -> Matrix Multiply/1
  Subsystem Aero. Coef. Rotation/1(C_L_A) -> Mux/1
  Subsystem Aero. Coef. Rotation/2(C_M_A) -> Mux/2
  Subsystem Aero. Coef. Rotation/3(C_N_A) -> Mux/3

== system Missile_Trim/Missle Model/Aerodynamics/Aerodynanamic Coefficents/Aerodynamics/Aerodynamic Coef. Translation ==
  Mach Number : Inport
  delta_eff : Inport  Port=2
  control inputs : Inport  Port=3
  alpha_t : Inport  Port=4
  phi_t : Inport  Port=5
  Constant2 : Constant  Value=0
  Matrix Multiply : Product  Multiplication=Matrix(*)
  Mux : Mux  Inputs=3
  Mux2 : Mux  Inputs=3
  Scope : Scope
  Subsystem Aero. Coef. Translation : Subsystem
  Transpose : Math  Commented=on  Operator=transpose  SaturateOnIntegerOverflow=on
  Wind Angles to Direction Cosine Matrix : aerolibtransform2/Wind Angles to  Direction Cosine Matrix
      settings: SourceProductName=Aerospace Blockset  SourceProductBaseCode=AE
  CX_CY_CZ : Outport
  CXa_CYa_CZa : Outport  Port=2
  wires:
  Mux/1 -> Matrix Multiply/2, CXa_CYa_CZa/1
  Matrix Multiply/1 -> CX_CY_CZ/1
  Mux2/1 -> Wind Angles to Direction Cosine Matrix/1
  phi_t/1 -> Mux2/1, Subsystem Aero. Coef. Translation/5(phi_t)
  Constant2/1 -> Mux2/2, Mux2/3
  Mach Number/1 -> Subsystem Aero. Coef. Translation/1(Mach number)
  control inputs/1 -> Subsystem Aero. Coef. Translation/4(control)
  alpha_t/1 -> Subsystem Aero. Coef. Translation/2(alpha_t)
  delta_eff/1 -> Subsystem Aero. Coef. Translation/3(delta_eff)
  Subsystem Aero. Coef. Translation/1(C_X_A) -> Scope/1, Mux/1
  Subsystem Aero. Coef. Translation/2(C_Y_A) -> Mux/2
  Subsystem Aero. Coef. Translation/3(C_Z_A) -> Mux/3
  Wind Angles to Direction Cosine Matrix/1 -> Matrix Multiply/1

== system Missile_Trim/Missle Model/Aerodynamics/Aerodynanamic Coefficents/Aerodynamics/Aerodynamic Coef. Rotation/Subsystem Aero. Coef. Rotation ==
  Mach Number : Inport
  alpha_t : Inport  Port=2
  phi_t : Inport  Port=3
  alpha_beta_V : Inport  Port=4
  PQR : Inport  Port=5
  control : Inport  Port=6
  C_X_C_Y_CZ : Inport  Port=7
  "Subsystem C_L_A " : Subsystem
  "Subsystem C_M_A " : Subsystem
  Subsystem C_N_A : Subsystem
  C_L_A : Outport
  C_M_A : Outport  Port=2
  C_N_A : Outport  Port=3
  wires:
  "Subsystem C_M_A "/1(C_M_A) -> C_M_A/1
  "Subsystem C_L_A "/1(C_L_A) -> C_L_A/1
  Subsystem C_N_A/1(C_N_A) -> C_N_A/1
  Mach Number/1 -> "Subsystem C_L_A "/1(Mach Number), "Subsystem C_M_A "/1(Mach Number), Subsystem C_N_A/1(Mach Number)
  alpha_t/1 -> Subsystem C_N_A/2(alpha_t), "Subsystem C_M_A "/2(alpha_t), "Subsystem C_L_A "/2(alpha_t)
  phi_t/1 -> Subsystem C_N_A/3(phi_t), "Subsystem C_M_A "/3(phi_t), "Subsystem C_L_A "/3(phi_t)
  alpha_beta_V/1 -> "Subsystem C_L_A "/4(alpha_beta_V), "Subsystem C_M_A "/4(alpha_beta_V), Subsystem C_N_A/4(alpha_beta_V)
  PQR/1 -> "Subsystem C_M_A "/5(PQR), "Subsystem C_L_A "/5(PQR), Subsystem C_N_A/5(PQR)
  control/1 -> "Subsystem C_M_A "/6(control), "Subsystem C_L_A "/6(control), Subsystem C_N_A/6(control)
  C_X_C_Y_CZ/1 -> "Subsystem C_M_A "/7(C_X_C_Y_C_Z), Subsystem C_N_A/7(C_X_C_Y_C_Z)

== system Missile_Trim/Missle Model/Aerodynamics/Aerodynanamic Coefficents/Aerodynamics/Aerodynamic Coef. Translation/Subsystem Aero. Coef. Translation ==
  Mach number : Inport
  alpha_t : Inport  Port=2
  delta_eff : Inport  Port=3
  control : Inport  Port=4
  phi_t : Inport  Port=5
  Subsystem C_X_A : Subsystem
  Subsystem C_Y_A : Subsystem
  Subsystem C_Z_A : Subsystem
  C_X_A : Outport
  C_Y_A : Outport  Port=2
  C_Z_A : Outport  Port=3
  wires:
  Subsystem C_X_A/1(C_X_A) -> C_X_A/1
  Subsystem C_Y_A/1(C_Y_A) -> C_Y_A/1
  Subsystem C_Z_A/1(C_Z_A) -> C_Z_A/1
  Mach number/1 -> Subsystem C_Z_A/1(Mach Number), Subsystem C_Y_A/1(Mach Number), Subsystem C_X_A/1(Mach Number)
  alpha_t/1 -> Subsystem C_Z_A/2(alpha_t), Subsystem C_Y_A/2(alpha_t), Subsystem C_X_A/2(alpha_t)
  delta_eff/1 -> Subsystem C_X_A/3(delta_eff)
  control/1 -> Subsystem C_Z_A/3(control), Subsystem C_Y_A/3(control)
  phi_t/1 -> Subsystem C_Z_A/4(phi_t), Subsystem C_Y_A/4(phi_t)

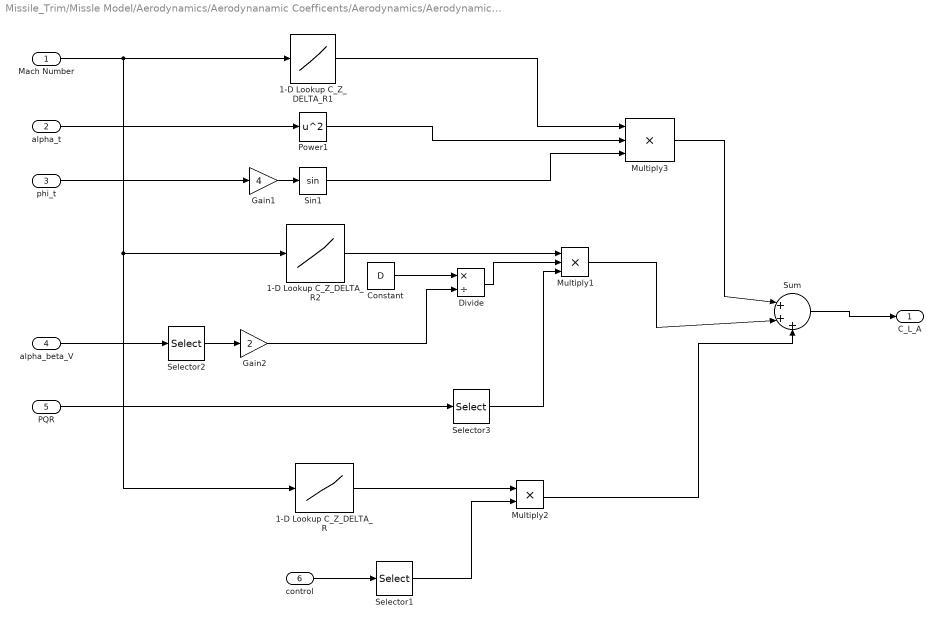
== system Missile_Trim/Missle Model/Aerodynamics/Aerodynanamic Coefficents/Aerodynamics/Aerodynamic Coef. Rotation/Subsystem Aero. Coef. Rotation/Subsystem C_L_A  ==
  Mach Number : Inport
  alpha_t : Inport  Port=2
  phi_t : Inport  Port=3
  alpha_beta_V : Inport  Port=4
  PQR : Inport  Port=5
  control : Inport  Port=6
  1-D Lookup C_Z_DELTA_R : Lookup_n-D  NumberOfTableDimensions=1  BreakpointsForDimension1=Tbl_MACH  Table=Tbl_CL_DEL_R  InternalRulePriority=Speed  RndMeth=Simplest  InputSameDT=on
  1-D Lookup C_Z_DELTA_R1 : Lookup_n-D  NumberOfTableDimensions=1  BreakpointsForDimension1=Tbl_MACH  Table=Tbl_CL_ALPHAT  InternalRulePriority=Speed  RndMeth=Simplest  InputSameDT=on
  1-D Lookup C_Z_DELTA_R2 : Lookup_n-D  NumberOfTableDimensions=1  BreakpointsForDimension1=Tbl_MACH  Table=Tbl_CL_P  InternalRulePriority=Speed  RndMeth=Simplest  InputSameDT=on
  Constant : Constant  Value=D
  Divide : Product  Inputs=*/
  Gain1 : Gain  Gain=4
  Gain2 : Gain  Gain=2
  Multiply1 : Product  Inputs=3
  Multiply2 : Product
  Multiply3 : Product  Inputs=3
  Power1 : Math  Operator=square  SaturateOnIntegerOverflow=on
  Selector1 : Selector  InputPortWidth=3  IndexOptions=Index vector (dialog)  Indices=[1]  OutputSizes=1
  Selector2 : Selector  InputPortWidth=3  IndexOptions=Index vector (dialog)  Indices=[3]  OutputSizes=1
  Selector3 : Selector  InputPortWidth=3  IndexOptions=Index vector (dialog)  Indices=[1]  OutputSizes=1
  Sin1 : Trigonometry
  Sum : Sum  Inputs=|+++
  C_L_A : Outport
  wires:
  1-D Lookup C_Z_DELTA_R1/1 -> Multiply3/1
  alpha_t/1 -> Power1/1
  Sum/1 -> C_L_A/1
  Mach Number/1 -> 1-D Lookup C_Z_DELTA_R/1, 1-D Lookup C_Z_DELTA_R2/1, 1-D Lookup C_Z_DELTA_R1/1
  1-D Lookup C_Z_DELTA_R2/1 -> Multiply1/1
  1-D Lookup C_Z_DELTA_R/1 -> Multiply2/1
  Multiply2/1 -> Sum/3
  Power1/1 -> Multiply3/2
  Sin1/1 -> Multiply3/3
  phi_t/1 -> Gain1/1
  Gain1/1 -> Sin1/1
  alpha_beta_V/1 -> Selector2/1
  Multiply3/1 -> Sum/1
  Multiply1/1 -> Sum/2
  Constant/1 -> Divide/1
  Selector2/1 -> Gain2/1
  Gain2/1 -> Divide/2
  Divide/1 -> Multiply1/2
  PQR/1 -> Selector3/1
  Selector3/1 -> Multiply1/3
  control/1 -> Selector1/1
  Selector1/1 -> Multiply2/2

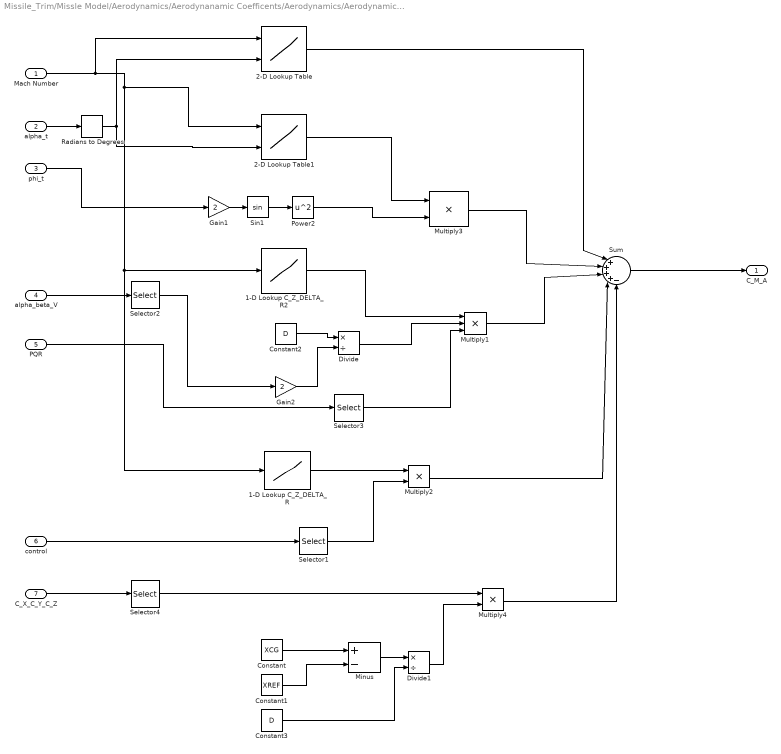
== system Missile_Trim/Missle Model/Aerodynamics/Aerodynanamic Coefficents/Aerodynamics/Aerodynamic Coef. Rotation/Subsystem Aero. Coef. Rotation/Subsystem C_M_A  ==
  Mach Number : Inport
  alpha_t : Inport  Port=2
  phi_t : Inport  Port=3
  alpha_beta_V : Inport  Port=4
  PQR : Inport  Port=5
  control : Inport  Port=6
  C_X_C_Y_C_Z : Inport  Port=7
  1-D Lookup C_Z_DELTA_R : Lookup_n-D  NumberOfTableDimensions=1  BreakpointsForDimension1=Tbl_MACH  Table=Tbl_CM_DEL_P  InternalRulePriority=Speed  RndMeth=Simplest  InputSameDT=on
  1-D Lookup C_Z_DELTA_R2 : Lookup_n-D  NumberOfTableDimensions=1  BreakpointsForDimension1=Tbl_MACH  Table=Tbl_CM_Q  DiagnosticForOutOfRangeInput=Warning  InternalRulePriority=Speed  RndMeth=Simplest  InputSameDT=on
  2-D Lookup Table : Lookup_n-D  BreakpointsForDimension1=Tbl_MACH  BreakpointsForDimension2=Tbl_ALPHAT  Table=Tbl_CM_0  DiagnosticForOutOfRangeInput=Warning  InternalRulePriority=Speed  RndMeth=Simplest  InputSameDT=on
  2-D Lookup Table1 : Lookup_n-D  BreakpointsForDimension1=Tbl_MACH  BreakpointsForDimension2=Tbl_ALPHAT  Table=Tbl_CM_PHIT  InternalRulePriority=Speed  RndMeth=Simplest  InputSameDT=on
  Constant : Constant  Value=XCG
  Constant1 : Constant  Value=XREF
  Constant2 : Constant  Value=D
  Constant3 : Constant  Value=D
  Divide : Product  Inputs=*/
  Divide1 : Product  Inputs=*/
  Gain1 : Gain  Gain=2
  Gain2 : Gain  Gain=2
  Minus : Sum  Inputs=+-
  Multiply1 : Product  Inputs=3
  Multiply2 : Product
  Multiply3 : Product
  Multiply4 : Product
  Power2 : Math  Operator=square  SaturateOnIntegerOverflow=on
  Radians to Degrees : simulink_extras/Transformations/Radians to Degrees
  Selector1 : Selector  InputPortWidth=3  IndexOptions=Index vector (dialog)  Indices=[2]  OutputSizes=1
  Selector2 : Selector  InputPortWidth=3  IndexOptions=Index vector (dialog)  Indices=[3]  OutputSizes=1
  Selector3 : Selector  InputPortWidth=3  IndexOptions=Index vector (dialog)  Indices=[2]  OutputSizes=1
  Selector4 : Selector  InputPortWidth=3  IndexOptions=Index vector (dialog)  Indices=[3]  OutputSizes=1
  Sin1 : Trigonometry
  Sum : Sum  Inputs=|++++-
  C_M_A : Outport
  wires:
  2-D Lookup Table/1 -> Sum/1
  Mach Number/1 -> 2-D Lookup Table/1, 2-D Lookup Table1/1, 1-D Lookup C_Z_DELTA_R/1, 1-D Lookup C_Z_DELTA_R2/1
  1-D Lookup C_Z_DELTA_R2/1 -> Multiply1/1
  1-D Lookup C_Z_DELTA_R/1 -> Multiply2/1
  Multiply2/1 -> Sum/4
  Sin1/1 -> Power2/1
  phi_t/1 -> Gain1/1
  Gain1/1 -> Sin1/1
  alpha_beta_V/1 -> Selector2/1
  Selector2/1 -> Gain2/1
  Gain2/1 -> Divide/2
  Divide/1 -> Multiply1/2
  PQR/1 -> Selector3/1
  Selector3/1 -> Multiply1/3
  control/1 -> Selector1/1
  Selector1/1 -> Multiply2/2
  2-D Lookup Table1/1 -> Multiply3/1
  Power2/1 -> Multiply3/2
  C_X_C_Y_C_Z/1 -> Selector4/1
  Constant/1 -> Minus/1
  Constant1/1 -> Minus/2
  Constant2/1 -> Divide/1
  Minus/1 -> Divide1/1
  Constant3/1 -> Divide1/2
  Selector4/1 -> Multiply4/1
  Divide1/1 -> Multiply4/2
  Multiply4/1 -> Sum/5
  Multiply1/1 -> Sum/3
  Multiply3/1 -> Sum/2
  alpha_t/1 -> Radians to Degrees/1
  Radians to Degrees/1 -> 2-D Lookup Table1/2, 2-D Lookup Table/2
  Sum/1 -> C_M_A/1

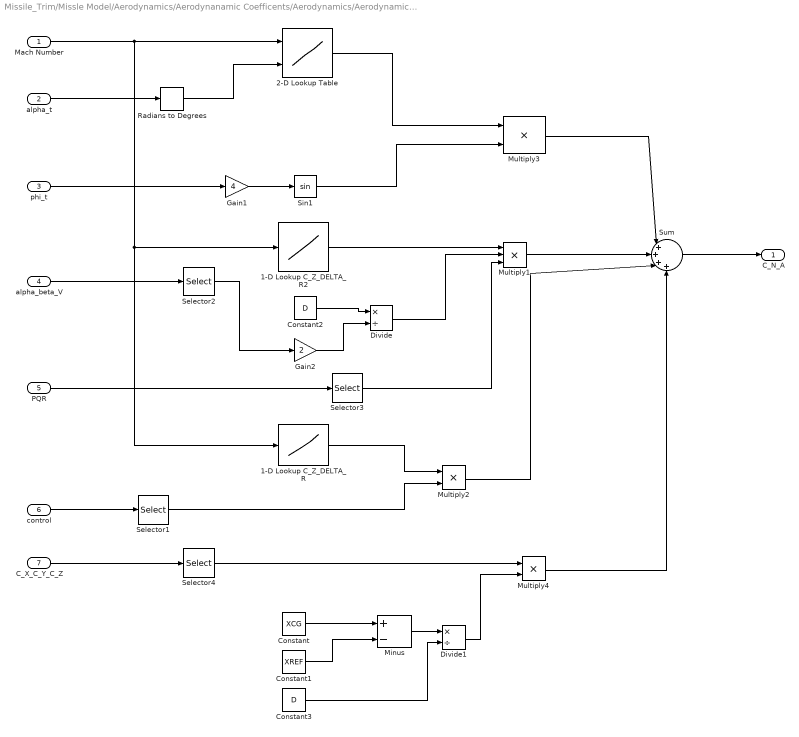
== system Missile_Trim/Missle Model/Aerodynamics/Aerodynanamic Coefficents/Aerodynamics/Aerodynamic Coef. Rotation/Subsystem Aero. Coef. Rotation/Subsystem C_N_A ==
  Mach Number : Inport
  alpha_t : Inport  Port=2
  phi_t : Inport  Port=3
  alpha_beta_V : Inport  Port=4
  PQR : Inport  Port=5
  control : Inport  Port=6
  C_X_C_Y_C_Z : Inport  Port=7
  1-D Lookup C_Z_DELTA_R : Lookup_n-D  NumberOfTableDimensions=1  BreakpointsForDimension1=Tbl_MACH  Table=Tbl_CN_DEL_Y  InternalRulePriority=Speed  RndMeth=Simplest  InputSameDT=on
  1-D Lookup C_Z_DELTA_R2 : Lookup_n-D  NumberOfTableDimensions=1  BreakpointsForDimension1=Tbl_MACH  Table=Tbl_CN_R  InternalRulePriority=Speed  RndMeth=Simplest  InputSameDT=on
  2-D Lookup Table : Lookup_n-D  BreakpointsForDimension1=Tbl_MACH  BreakpointsForDimension2=Tbl_ALPHAT  Table=Tbl_CN_PHIT  InternalRulePriority=Speed  RndMeth=Simplest  InputSameDT=on
  Constant : Constant  Value=XCG
  Constant1 : Constant  Value=XREF
  Constant2 : Constant  Value=D
  Constant3 : Constant  Value=D
  Divide : Product  Inputs=*/
  Divide1 : Product  Inputs=*/
  Gain1 : Gain  Gain=4
  Gain2 : Gain  Gain=2
  Minus : Sum  Inputs=+-
  Multiply1 : Product  Inputs=3
  Multiply2 : Product
  Multiply3 : Product
  Multiply4 : Product
  Radians to Degrees : simulink_extras/Transformations/Radians to Degrees
  Selector1 : Selector  InputPortWidth=3  IndexOptions=Index vector (dialog)  Indices=[3]  OutputSizes=1
  Selector2 : Selector  InputPortWidth=3  IndexOptions=Index vector (dialog)  Indices=[3]  OutputSizes=1
  Selector3 : Selector  InputPortWidth=3  IndexOptions=Index vector (dialog)  Indices=[3]  OutputSizes=1
  Selector4 : Selector  InputPortWidth=3  IndexOptions=Index vector (dialog)  Indices=[2]  OutputSizes=1
  Sin1 : Trigonometry
  Sum : Sum  Inputs=|++++
  C_N_A : Outport
  wires:
  2-D Lookup Table/1 -> Multiply3/1
  alpha_t/1 -> Radians to Degrees/1
  Sum/1 -> C_N_A/1
  Mach Number/1 -> 2-D Lookup Table/1, 1-D Lookup C_Z_DELTA_R/1, 1-D Lookup C_Z_DELTA_R2/1
  1-D Lookup C_Z_DELTA_R2/1 -> Multiply1/1
  1-D Lookup C_Z_DELTA_R/1 -> Multiply2/1
  Multiply2/1 -> Sum/3
  Sin1/1 -> Multiply3/2
  phi_t/1 -> Gain1/1
  Gain1/1 -> Sin1/1
  alpha_beta_V/1 -> Selector2/1
  Selector2/1 -> Gain2/1
  Divide/1 -> Multiply1/2
  PQR/1 -> Selector3/1
  Selector3/1 -> Multiply1/3
  control/1 -> Selector1/1
  Selector1/1 -> Multiply2/2
  C_X_C_Y_C_Z/1 -> Selector4/1
  Constant/1 -> Minus/1
  Constant1/1 -> Minus/2
  Constant2/1 -> Divide/1
  Minus/1 -> Divide1/1
  Constant3/1 -> Divide1/2
  Selector4/1 -> Multiply4/1
  Divide1/1 -> Multiply4/2
  Multiply4/1 -> Sum/4
  Multiply1/1 -> Sum/2
  Multiply3/1 -> Sum/1
  Radians to Degrees/1 -> 2-D Lookup Table/2
  Gain2/1 -> Divide/2

== system Missile_Trim/Missle Model/Aerodynamics/Aerodynanamic Coefficents/Aerodynamics/Aerodynamic Coef. Translation/Subsystem Aero. Coef. Translation/Subsystem C_X_A ==
  Mach Number : Inport
  alpha_t : Inport  Port=2
  delta_eff : Inport  Port=3
  1-D Lookup C_X_0 : Lookup_n-D  NumberOfTableDimensions=1  BreakpointsForDimension1=Tbl_MACH  Table=Tbl_CX_0  DiagnosticForOutOfRangeInput=Warning  InternalRulePriority=Speed  RndMeth=Simplest  InputSameDT=on
  1-D Lookup C_X_ALPHA_T : Lookup_n-D  NumberOfTableDimensions=1  BreakpointsForDimension1=Tbl_MACH  BeginIndexSearchUsingPreviousIndexResult=on  Table=Tbl_CX_ALPHAT  DiagnosticForOutOfRangeInput=Warning  InternalRulePriority=Speed  RndMeth=Simplest  InputSameDT=on
  1-D Lookup C_X_DELTA_EFF : Lookup_n-D  NumberOfTableDimensions=1  BreakpointsForDimension1=Tbl_MACH  Table=Tbl_CX_DEL_EFF  DiagnosticForOutOfRangeInput=Warning  InternalRulePriority=Speed  RndMeth=Simplest  InputSameDT=on
  Display : Display
  Multiply : Product
  Multiply1 : Product
  Scope : Scope
  Square : Math  Operator=square  SaturateOnIntegerOverflow=on
  Sum : Sum  Inputs=|+++
  C_X_A : Outport
  wires:
  Multiply/1 -> Sum/2
  Multiply1/1 -> Display/1, Sum/3
  1-D Lookup C_X_DELTA_EFF/1 -> Multiply1/1
  1-D Lookup C_X_ALPHA_T/1 -> Multiply/1
  1-D Lookup C_X_0/1 -> Sum/1
  Mach Number/1 -> 1-D Lookup C_X_DELTA_EFF/1, 1-D Lookup C_X_ALPHA_T/1, Scope/1, 1-D Lookup C_X_0/1
  Sum/1 -> C_X_A/1
  alpha_t/1 -> Multiply/2
  delta_eff/1 -> Square/1
  Square/1 -> Multiply1/2

== system Missile_Trim/Missle Model/Aerodynamics/Aerodynanamic Coefficents/Aerodynamics/Aerodynamic Coef. Translation/Subsystem Aero. Coef. Translation/Subsystem C_Y_A ==
  Mach Number : Inport
  alpha_t : Inport  Port=2
  control : Inport  Port=3
  phi_t : Inport  Port=4
  1-D Lookup C_Y_DELTA_Y : Lookup_n-D  NumberOfTableDimensions=1  BreakpointsForDimension1=Tbl_MACH  Table=Tbl_CY_DEL_Y  DiagnosticForOutOfRangeInput=Warning  InternalRulePriority=Speed  RndMeth=Simplest  InputSameDT=on
  2-D Lookup CY_PHIT : Lookup_n-D  BreakpointsForDimension1=Tbl_MACH  BreakpointsForDimension2=Tbl_ALPHAT  Table=Tbl_CY_PHIT  DiagnosticForOutOfRangeInput=Warning  InternalRulePriority=Speed  RndMeth=Simplest  InputSameDT=on
  Gain : Gain  Gain=4
  Multiply1 : Product
  Multiply2 : Product
  Radians to Degrees : simulink_extras/Transformations/Radians to Degrees
  Sin : Trigonometry
  Sum : Sum  Inputs=|++
  delta_y : Selector  InputPortWidth=3  IndexOptions=Index vector (dialog)  Indices=[3]  OutputSizes=1
  C_Y_A : Outport
  wires:
  Multiply1/1 -> Sum/2
  1-D Lookup C_Y_DELTA_Y/1 -> Multiply1/1
  2-D Lookup CY_PHIT/1 -> Multiply2/1
  Mach Number/1 -> 1-D Lookup C_Y_DELTA_Y/1, 2-D Lookup CY_PHIT/1
  Sum/1 -> C_Y_A/1
  Gain/1 -> Sin/1
  phi_t/1 -> Gain/1
  control/1 -> delta_y/1
  alpha_t/1 -> Radians to Degrees/1
  delta_y/1 -> Multiply1/2
  Sin/1 -> Multiply2/2
  Multiply2/1 -> Sum/1
  Radians to Degrees/1 -> 2-D Lookup CY_PHIT/2

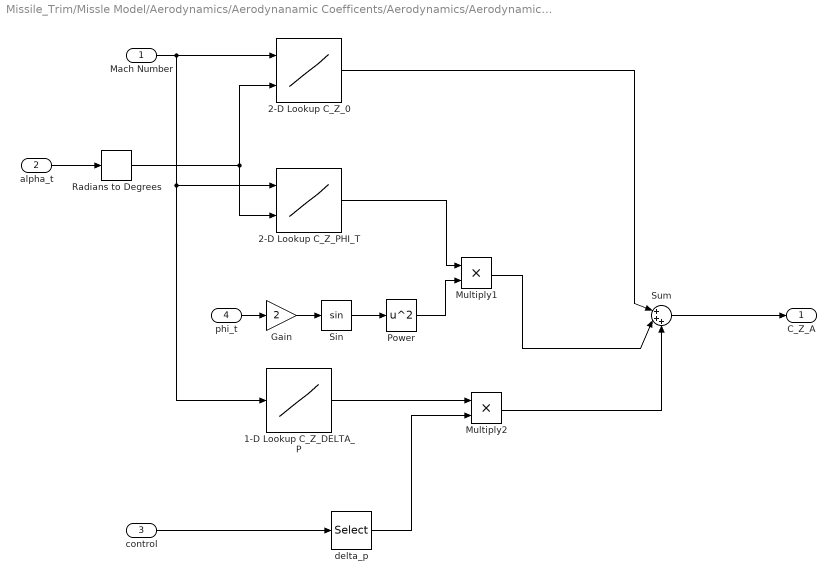
== system Missile_Trim/Missle Model/Aerodynamics/Aerodynanamic Coefficents/Aerodynamics/Aerodynamic Coef. Translation/Subsystem Aero. Coef. Translation/Subsystem C_Z_A ==
  Mach Number : Inport
  alpha_t : Inport  Port=2
  control : Inport  Port=3
  phi_t : Inport  Port=4
  1-D Lookup C_Z_DELTA_P : Lookup_n-D  NumberOfTableDimensions=1  BreakpointsForDimension1=Tbl_MACH  Table=Tbl_CZ_DEL_P  InternalRulePriority=Speed  RndMeth=Simplest  InputSameDT=on
  2-D Lookup C_Z_0 : Lookup_n-D  BreakpointsForDimension1=Tbl_MACH  BreakpointsForDimension2=Tbl_ALPHAT  Table=Tbl_CZ_0  DiagnosticForOutOfRangeInput=Warning  InternalRulePriority=Speed  RndMeth=Simplest  InputSameDT=on
  2-D Lookup C_Z_PHI_T : Lookup_n-D  BreakpointsForDimension1=Tbl_MACH  BreakpointsForDimension2=Tbl_ALPHAT  Table=Tbl_CZ_PHIT  InternalRulePriority=Speed  RndMeth=Simplest  InputSameDT=on
  Gain : Gain  Gain=2
  Multiply1 : Product
  Multiply2 : Product
  Power : Math  Operator=square  SaturateOnIntegerOverflow=on
  Radians to Degrees : simulink_extras/Transformations/Radians to Degrees
  Sin : Trigonometry
  Sum : Sum  Inputs=|+++
  delta_p : Selector  InputPortWidth=3  IndexOptions=Index vector (dialog)  Indices=[2]  OutputSizes=1
  C_Z_A : Outport
  wires:
  2-D Lookup C_Z_0/1 -> Sum/1
  delta_p/1 -> Multiply2/2
  alpha_t/1 -> Radians to Degrees/1
  control/1 -> delta_p/1
  Sum/1 -> C_Z_A/1
  Mach Number/1 -> 2-D Lookup C_Z_PHI_T/1, 1-D Lookup C_Z_DELTA_P/1, 2-D Lookup C_Z_0/1
  2-D Lookup C_Z_PHI_T/1 -> Multiply1/1
  Multiply1/1 -> Sum/2
  Gain/1 -> Sin/1
  phi_t/1 -> Gain/1
  Sin/1 -> Power/1
  Power/1 -> Multiply1/2
  1-D Lookup C_Z_DELTA_P/1 -> Multiply2/1
  Multiply2/1 -> Sum/3
  Radians to Degrees/1 -> 2-D Lookup C_Z_0/2, 2-D Lookup C_Z_PHI_T/2
